simulink model "State_Space_Quadrotor"  (Simulink 7.7)
settings: Solver=ode45  StartTime=0.0  StopTime=3  RelTol=1e-3
undefined symbols (not defined in the file or in its folder): quad
libraries: simulink x4
settings Model: Creator=Alexey  LastModifiedBy=Alexey

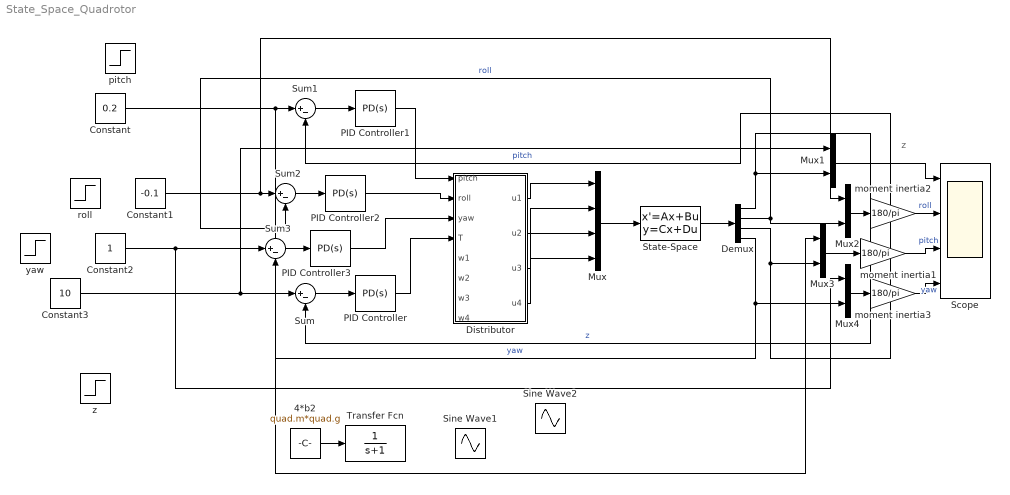
== system State_Space_Quadrotor ==
  note: z
  4*b2 : Constant  Value=quad.m*quad.g
  Constant : Constant  Value=0.2
  Constant1 : Constant  Value=-0.1
  Constant2 : Constant
  Constant3 : Constant  Value=10
  Demux : Demux
  Distributor : Subsystem
  Mux : Mux
  Mux{1..4} (4 alike) : Mux  Inputs=2
  PID Controller : simulink/Continuous/PID Controller  SystemSampleTime=-1  Controller=PD  TimeDomain=Continuous-time  SampleTime=1  IntegratorMethod=Forward Euler  FilterMethod=Forward Euler  Form=Parallel  P=50  I=0  D=10  N=100  InitialConditionSource=internal  InitialConditionForIntegrator=0  InitialConditionForFilter=0  ExternalReset=none  LimitOutput=off  UpperSaturationLimit=inf  LowerSaturationLimit=-inf  LinearizeAsGain=off  AntiWindupMode=none  Kb=1  TrackingMode=off  Kt=1  PParamMin=[]  PParamMax=[]  IParamMin=[]  IParamMax=[]  DParamMin=[]  DParamMax=[]  NParamMin=[]  NParamMax=[]  KbParamMin=[]  KbParamMax=[]  KtParamMin=[]  KtParamMax=[]  POutMin=[]  POutMax=[]  IOutMin=[]  IOutMax=[]  DOutMin=[]  DOutMax=[]  NOutMin=[]  NOutMax=[]  KbOutMin=[]  KbOutMax=[]  KtOutMin=[]  KtOutMax=[]  IntegratorOutMin=[]  IntegratorOutMax=[]  FilterOutMin=[]  FilterOutMax=[]  SumOutMin=[]  SumOutMax=[]  SumI1OutMin=[]  SumI1OutMax=[]  SumI2OutMin=[]  SumI2OutMax=[]  SumI3OutMin=[]  SumI3OutMax=[]  SumDOutMin=[]  SumDOutMax=[]  SaturationOutMin=[]  SaturationOutMax=[]  IntegratorContinuousStateAttributes=''  IntegratorStateMustResolveToSignalObject=off  IntegratorRTWStateStorageClass=Auto  FilterContinuousStateAttributes=''  FilterStateMustResolveToSignalObject=off  FilterRTWStateStorageClass=Auto
  PID Controller1 : simulink/Continuous/PID Controller  SystemSampleTime=-1  Controller=PD  TimeDomain=Continuous-time  SampleTime=1  IntegratorMethod=Forward Euler  FilterMethod=Forward Euler  Form=Parallel  P=0.1  I=0  D=0.4  N=100  InitialConditionSource=internal  InitialConditionForIntegrator=0  InitialConditionForFilter=0  ExternalReset=none  LimitOutput=off  UpperSaturationLimit=inf  LowerSaturationLimit=-inf  LinearizeAsGain=off  AntiWindupMode=none  Kb=1  TrackingMode=off  Kt=1  PParamMin=[]  PParamMax=[]  IParamMin=[]  IParamMax=[]  DParamMin=[]  DParamMax=[]  NParamMin=[]  NParamMax=[]  KbParamMin=[]  KbParamMax=[]  KtParamMin=[]  KtParamMax=[]  POutMin=[]  POutMax=[]  IOutMin=[]  IOutMax=[]  DOutMin=[]  DOutMax=[]  NOutMin=[]  NOutMax=[]  KbOutMin=[]  KbOutMax=[]  KtOutMin=[]  KtOutMax=[]  IntegratorOutMin=[]  IntegratorOutMax=[]  FilterOutMin=[]  FilterOutMax=[]  SumOutMin=[]  SumOutMax=[]  SumI1OutMin=[]  SumI1OutMax=[]  SumI2OutMin=[]  SumI2OutMax=[]  SumI3OutMin=[]  SumI3OutMax=[]  SumDOutMin=[]  SumDOutMax=[]  SaturationOutMin=[]  SaturationOutMax=[]  IntegratorContinuousStateAttributes=''  IntegratorStateMustResolveToSignalObject=off  IntegratorRTWStateStorageClass=Auto  FilterContinuousStateAttributes=''  FilterStateMustResolveToSignalObject=off  FilterRTWStateStorageClass=Auto
  PID Controller2 : simulink/Continuous/PID Controller  SystemSampleTime=-1  Controller=PD  TimeDomain=Continuous-time  SampleTime=1  IntegratorMethod=Forward Euler  FilterMethod=Forward Euler  Form=Parallel  P=0.1  I=0  D=0.5  N=100  InitialConditionSource=internal  InitialConditionForIntegrator=0  InitialConditionForFilter=0  ExternalReset=none  LimitOutput=off  UpperSaturationLimit=inf  LowerSaturationLimit=-inf  LinearizeAsGain=off  AntiWindupMode=none  Kb=1  TrackingMode=off  Kt=1  PParamMin=[]  PParamMax=[]  IParamMin=[]  IParamMax=[]  DParamMin=[]  DParamMax=[]  NParamMin=[]  NParamMax=[]  KbParamMin=[]  KbParamMax=[]  KtParamMin=[]  KtParamMax=[]  POutMin=[]  POutMax=[]  IOutMin=[]  IOutMax=[]  DOutMin=[]  DOutMax=[]  NOutMin=[]  NOutMax=[]  KbOutMin=[]  KbOutMax=[]  KtOutMin=[]  KtOutMax=[]  IntegratorOutMin=[]  IntegratorOutMax=[]  FilterOutMin=[]  FilterOutMax=[]  SumOutMin=[]  SumOutMax=[]  SumI1OutMin=[]  SumI1OutMax=[]  SumI2OutMin=[]  SumI2OutMax=[]  SumI3OutMin=[]  SumI3OutMax=[]  SumDOutMin=[]  SumDOutMax=[]  SaturationOutMin=[]  SaturationOutMax=[]  IntegratorContinuousStateAttributes=''  IntegratorStateMustResolveToSignalObject=off  IntegratorRTWStateStorageClass=Auto  FilterContinuousStateAttributes=''  FilterStateMustResolveToSignalObject=off  FilterRTWStateStorageClass=Auto
  PID Controller3 : simulink/Continuous/PID Controller  SystemSampleTime=-1  Controller=PD  TimeDomain=Continuous-time  SampleTime=1  IntegratorMethod=Forward Euler  FilterMethod=Forward Euler  Form=Parallel  P=1  I=0  D=4  N=100  InitialConditionSource=internal  InitialConditionForIntegrator=0  InitialConditionForFilter=0  ExternalReset=none  LimitOutput=off  UpperSaturationLimit=inf  LowerSaturationLimit=-inf  LinearizeAsGain=off  AntiWindupMode=none  Kb=1  TrackingMode=off  Kt=1  PParamMin=[]  PParamMax=[]  IParamMin=[]  IParamMax=[]  DParamMin=[]  DParamMax=[]  NParamMin=[]  NParamMax=[]  KbParamMin=[]  KbParamMax=[]  KtParamMin=[]  KtParamMax=[]  POutMin=[]  POutMax=[]  IOutMin=[]  IOutMax=[]  DOutMin=[]  DOutMax=[]  NOutMin=[]  NOutMax=[]  KbOutMin=[]  KbOutMax=[]  KtOutMin=[]  KtOutMax=[]  IntegratorOutMin=[]  IntegratorOutMax=[]  FilterOutMin=[]  FilterOutMax=[]  SumOutMin=[]  SumOutMax=[]  SumI1OutMin=[]  SumI1OutMax=[]  SumI2OutMin=[]  SumI2OutMax=[]  SumI3OutMin=[]  SumI3OutMax=[]  SumDOutMin=[]  SumDOutMax=[]  SaturationOutMin=[]  SaturationOutMax=[]  IntegratorContinuousStateAttributes=''  IntegratorStateMustResolveToSignalObject=off  IntegratorRTWStateStorageClass=Auto  FilterContinuousStateAttributes=''  FilterStateMustResolveToSignalObject=off  FilterRTWStateStorageClass=Auto
  Scope : Scope  NumInputPorts=4
      settings: TimeRange=2  YMin=-500~0~-1~-225  YMax=100~800~1~-75
  Sine Wave1 : Sin  Amplitude=100000  Frequency=0.5  SampleTime=0
  Sine Wave2 : Sin  Amplitude=10000000  SampleTime=0
  State-Space : StateSpace  A=|  B=|  C=|  D=|
      A=|
      | [0     0     0     0     0     0     0     0;
      |      0     0     0     0     0     0     0     0;
      |      0     0     0     0     0     0     0     0;
      |      0     0     0     0     0     0     0     0;
      |      1     0     0     0     0     0     0     0;
      |      0     1     0     0     0     0     0     0;
      |      0     0     1     0     0     0     0     0;
      |      0     0     0     1     0     0     0     0
      | ]
      B=|
      | [1/quad.m*quad.b     0     0     0;
      |      0     0     1/quad.Ixx*quad.b*quad.l     0;
      |      0     0     0     1/quad.Iyy*quad.b*quad.l;
      |      0     1/quad.Izz*quad.k*quad.r     0     0;
      |      0     0     0     0;
      |      0     0     0     0;
      |      0     0     0     0;
      |      0     0     0     0
      | ]
      C=|
      | [0     0     0     0     1     0     0     0;
      |      0     0     0     0     0     1     0     0;
      |      0     0     0     0     0     0     1     0;
      |      0     0     0     0     0     0     0     1
      | ]
      D=|
      | [[0     0     0     0;
      |      0     0     0     0;
      |      0     0     0     0;
      |      0     0     0     0]]
  Sum{,1..3} (4 alike) : Sum  Inputs=|+-
  Transfer Fcn : TransferFcn  Denominator=[1 1]
  moment inertia1 : Gain  Gain=180/pi
  moment inertia2 : Gain  Gain=180/pi
  moment inertia3 : Gain  Gain=180/pi
  pitch : Step  Time=3.5  After=-0.1  SampleTime=0
  roll : Step  Time=3  Before=-0.2  After=0.1  SampleTime=0
  yaw : Step  Time=2  After=2  SampleTime=0
  z : Step  Time=0  After=10  SampleTime=0
  wires:
  State-Space/1 -> Demux/1
  Demux/1 -> Mux1/2, Sum/2  "z"
  Demux/2 -> Sum2/2, Mux2/2  "roll"
  Demux/3 -> Sum1/2, Mux3/2  "pitch"
  Demux/4 -> Sum3/2, Mux4/2  "yaw"
  Mux/1 -> State-Space/1
  Distributor/2("u2 ") -> Mux/2
  Distributor/3("u3 ") -> Mux/3
  Distributor/4("u4 ") -> Mux/4
  Sum/1 -> PID Controller/1
  Constant3/1 -> Sum/1, Mux1/1
  PID Controller/1 -> Distributor/4(T)
  Constant/1 -> Sum1/1, Mux3/1
  Sum1/1 -> PID Controller1/1
  PID Controller1/1 -> Distributor/1(pitch)
  PID Controller2/1 -> Distributor/2(roll)
  Sum2/1 -> PID Controller2/1
  PID Controller3/1 -> Distributor/3(yaw)
  Sum3/1 -> PID Controller3/1
  Constant2/1 -> Mux4/1, Sum3/1
  Constant1/1 -> Sum2/1, Mux2/1
  Mux1/1 -> Scope/1
  Mux2/1 -> moment inertia2/1
  Mux3/1 -> moment inertia1/1
  Mux4/1 -> moment inertia3/1
  Distributor/1("u1 ") -> Mux/1
  4*b2/1 -> Transfer Fcn/1
  moment inertia2/1 -> Scope/2  "roll"
  moment inertia1/1 -> Scope/3  "pitch"
  moment inertia3/1 -> Scope/4  "yaw"
  ? -> Distributor/8(w4), Distributor/7(w3), Distributor/6(w2), Distributor/5(w1)

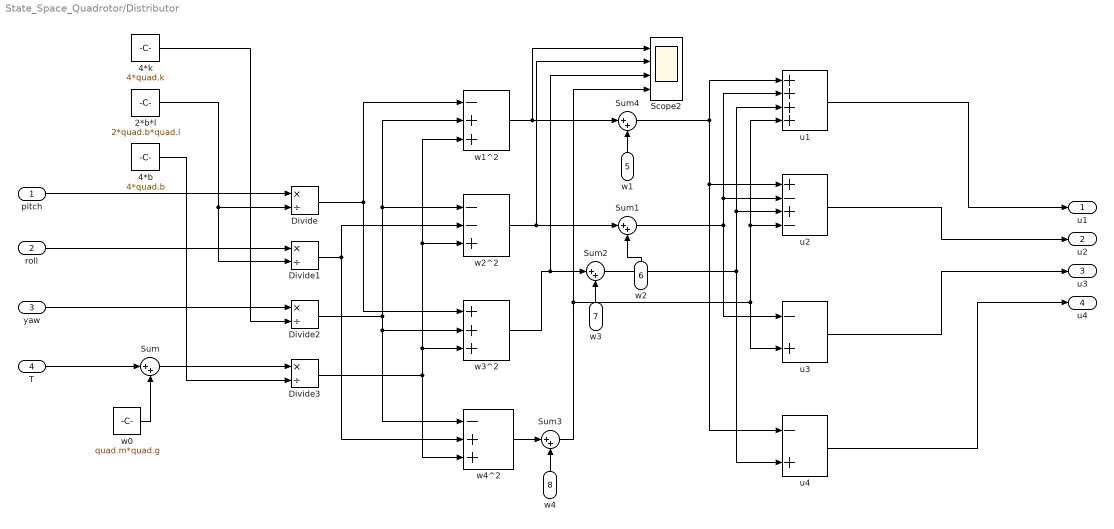
== system State_Space_Quadrotor/Distributor ==
  pitch : Inport
  roll : Inport  Port=2
  yaw : Inport  Port=3
  T : Inport  Port=4
  w1 : Inport  Port=5
  w2 : Inport  Port=6
  w3 : Inport  Port=7
  w4 : Inport  Port=8
  2*b*l : Constant  Value=2*quad.b*quad.l
  4*b : Constant  Value=4*quad.b
  4*k : Constant  Value=4*quad.k
  Divide{,1..3} (4 alike) : Product  Inputs=*/
  Scope2 : Scope  NumInputPorts=4
      settings: YMin=-1.5e+007~-2.5e+006~-1.5e+007~-2.5e+006  YMax=2.5e+006~1.25e+007~2.5e+006~1.25e+007  SaveName=ScopeData9
  Sum{,1..4} (5 alike) : Sum  Inputs=|++
  u1 : Sum  Inputs=++++
  u2 : Sum  Inputs=+-+-
  u3 : Sum  Inputs=-+
  u4 : Sum  Inputs=-+
  w0 : Constant  Value=quad.m*quad.g
  w1^2 : Sum  Inputs=-++
  w2^2 : Sum  Inputs=--+
  w3^2 : Sum  Inputs=+++
  w4^2 : Sum  Inputs=-++
  "u1 " : Outport
  "u2 " : Outport  Port=2
  "u3 " : Outport  Port=3
  "u4 " : Outport  Port=4
  wires:
  4*k/1 -> Divide2/2
  Divide1/1 -> w2^2/2, w4^2/2
  Divide2/1 -> w3^2/2, w4^2/1, w1^2/2, w2^2/1
  Divide/1 -> w1^2/1, w3^2/1
  4*b/1 -> Divide3/2
  yaw/1 -> Divide2/1
  2*b*l/1 -> Divide/2, Divide1/2
  roll/1 -> Divide1/1
  pitch/1 -> Divide/1
  Sum4/1 -> u1/1, u2/1, u4/1
  Sum1/1 -> u1/2, u2/2, u3/1
  Sum2/1 -> u1/3, u2/3, u4/2
  Sum3/1 -> Scope2/4, u1/4, u2/4, u3/2
  Divide3/1 -> w1^2/3, w2^2/3, w3^2/3, w4^2/3
  u1/1 -> "u1 "/1
  u2/1 -> "u2 "/1
  u3/1 -> "u3 "/1
  u4/1 -> "u4 "/1
  T/1 -> Sum/1
  Sum/1 -> Divide3/1
  w0/1 -> Sum/2
  w1^2/1 -> Sum4/1, Scope2/1
  w1/1 -> Sum4/2
  w2/1 -> Sum1/2
  w3/1 -> Sum2/2
  w4/1 -> Sum3/2
  w2^2/1 -> Sum1/1, Scope2/2
  w3^2/1 -> Sum2/1, Scope2/3
  w4^2/1 -> Sum3/1
